simulink model "ThreeDof_2015_11_21"  (R2013a)
settings: Solver=ode45  StartTime=0.0  StopTime=100  RelTol=1e-3
undefined symbols (not defined in the file): cbar, Earth, F, Light, MIL, MSSN, statdyn, WGS84
libraries: aerolibwind2 x3, aerolibtransform2 x3, aerolibasang x3, aerolibactuator x3, aerolibobsolete x2, aerolibconvert2 x2, aerolibatmos2 x1, PowerFlowLib x1, simulink x1, aerolib3dof2 x1, aerolibadyn x1
settings Model: Creator=mwillms4  LastModifiedBy=ASELab1

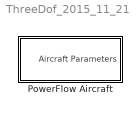
== system ThreeDof_2015_11_21 ==
  PowerFlow Aircraft : Subsystem

== system ThreeDof_2015_11_21/PowerFlow Aircraft ==
  Bus Selector : BusSelector  OutputSignals=alt
  Environment : Subsystem  TreatAsAtomicUnit=on
  Mission Profile : PowerFlowLib/Mission Profile/Mission Profile  mssn_check=off  mssn_prof=MSSN  del_P=0  del_T=0  del_rho=0  pres_msl=101.3  temp_msl=15  dens_msl=1.229
  Pilot : Subsystem  TreatAsAtomicUnit=on
  Scope : Scope
  Vehicle System Model : Subsystem
  Aircraft Parameters : Outport
  wires:
  Environment/1(Env) -> Vehicle System Model/1(Env)
  Pilot/1(cmd) -> Vehicle System Model/2(Pilot)
  Mission Profile/1 -> Pilot/2(Mission Profile)
  Vehicle System Model/1(PlantData) -> Aircraft Parameters/1, Environment/1(plant), Pilot/1(Aircraft), Bus Selector/1
  Bus Selector/1 -> Scope/1  "<alt>"

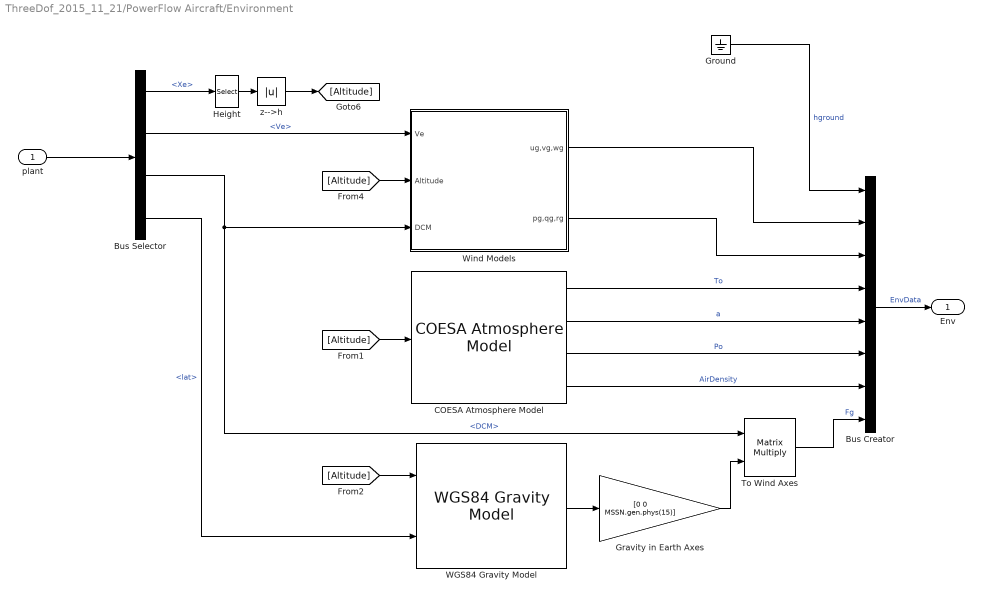
== system ThreeDof_2015_11_21/PowerFlow Aircraft/Environment ==
  plant : Inport
  Bus Creator : BusCreator  Inputs='hground','WindVelocity','WindAngularRates','To','a','Po','AirDensity','Fg'
  Bus Selector : BusSelector  OutputSignals=Xe,Ve,DCM,lat
  COESA Atmosphere Model : aerolibatmos2/COESA Atmosphere Model  units=Metric (MKS)  spec=1976 COESA-extended U.S. Standard Atmosphere  model=Profile  profile_var=High temperature  profile_percent=1%  profile_alt=5 km (16404 ft)  envelope_var=High temperature  envelope_percent=1%  action=Warning
  Gravity in Earth Axes : Gain  Gain=[0 0 MSSN.gen.phys(15)]  SaturateOnIntegerOverflow=on  OutDataTypeStr=Inherit: Same as input  ParamDataTypeStr=Inherit: Same as input
  Ground : Ground
  Height : Selector  IndexMode=Zero-based  InputPortWidth=3  IndexOptions=Index vector (dialog)  Indices=2  OutputSizes=1
  To Wind Axes : Product  Multiplication=Matrix(*)  SaturateOnIntegerOverflow=on  InputSameDT=on  OutDataTypeStr=Inherit: Same as first input
  WGS84 Gravity Model : aerolibobsolete/WGS84 Gravity Model  model=WGS84 Taylor Series  units=Metric (MKS)  no_atmos=on  precessing=on  month=February  day=1  year=2000  no_centrifugal=on  action=Warning
  Wind Models : Subsystem
  z-->h : Abs  SaturateOnIntegerOverflow=on
  Env : Outport  InitialOutput=0
  wires:
  Bus Selector/3 -> Wind Models/3(DCM), To Wind Axes/1  "<DCM>"
  Bus Selector/2 -> Wind Models/1(Ve)  "<Ve>"
  Bus Selector/1 -> Height/1  "<Xe>"
  [Altitude] -> COESA Atmosphere Model/1
  [Altitude] -> WGS84 Gravity Model/1
  [Altitude] -> Wind Models/2(Altitude)
  z-->h/1 -> [Altitude]
  plant/1 -> Bus Selector/1
  Bus Creator/1 -> Env/1  "EnvData"
  To Wind Axes/1 -> Bus Creator/8  "Fg"
  Gravity in Earth Axes/1 -> To Wind Axes/2
  WGS84 Gravity Model/1 -> Gravity in Earth Axes/1
  Bus Selector/4 -> WGS84 Gravity Model/2  "<lat>"
  Height/1 -> z-->h/1
  COESA Atmosphere Model/1 -> Bus Creator/4  "To"
  COESA Atmosphere Model/3 -> Bus Creator/6  "Po"
  COESA Atmosphere Model/2 -> Bus Creator/5  "a"
  COESA Atmosphere Model/4 -> Bus Creator/7  "AirDensity"
  Wind Models/2(pg,qg,rg) -> Bus Creator/3
  Wind Models/1(ug,vg,wg) -> Bus Creator/2
  Ground/1 -> Bus Creator/1  "hground"

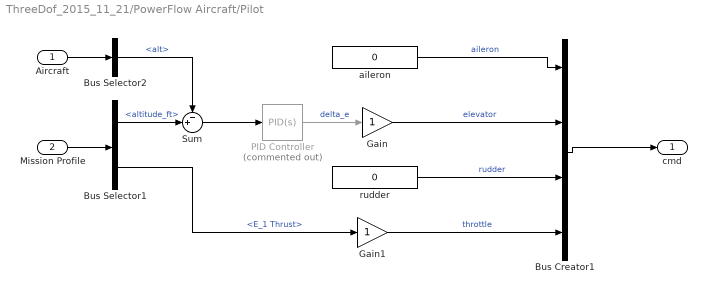
== system ThreeDof_2015_11_21/PowerFlow Aircraft/Pilot ==
  Aircraft : Inport
  Mission Profile : Inport  Port=2
  Bus Creator1 : BusCreator
  Bus Selector1 : BusSelector  OutputSignals=Flight parameters.altitude_ft,Engines.E_1 Thrust
  Bus Selector2 : BusSelector  OutputSignals=alt
  Gain : Gain
  Gain1 : Gain
  PID Controller : simulink/Continuous/PID Controller  Commented=on  Controller=PID  TimeDomain=Continuous-time  SampleTime=1  IntegratorMethod=Forward Euler  FilterMethod=Forward Euler  Form=Parallel  P=1  I=1  D=0  N=100  InitialConditionSource=internal  InitialConditionForIntegrator=0  InitialConditionForFilter=0  ExternalReset=none  LimitOutput=off  UpperSaturationLimit=inf  LowerSaturationLimit=-inf  LinearizeAsGain=on  AntiWindupMode=none  Kb=1  TrackingMode=off  Kt=1  PParamMin=[]  PParamMax=[]  IParamMin=[]  IParamMax=[]  DParamMin=[]  DParamMax=[]  NParamMin=[]  NParamMax=[]  KbParamMin=[]  KbParamMax=[]  KtParamMin=[]  KtParamMax=[]  POutMin=[]  POutMax=[]  IOutMin=[]  IOutMax=[]  DOutMin=[]  DOutMax=[]  NOutMin=[]  NOutMax=[]  KbOutMin=[]  KbOutMax=[]  KtOutMin=[]  KtOutMax=[]  IntegratorOutMin=[]  IntegratorOutMax=[]  FilterOutMin=[]  FilterOutMax=[]  SumOutMin=[]  SumOutMax=[]  SumI1OutMin=[]  SumI1OutMax=[]  SumI2OutMin=[]  SumI2OutMax=[]  SumI3OutMin=[]  SumI3OutMax=[]  SumDOutMin=[]  SumDOutMax=[]  SaturationOutMin=[]  SaturationOutMax=[]  IntegratorContinuousStateAttributes=''  IntegratorStateMustResolveToSignalObject=off  IntegratorRTWStateStorageClass=Auto  FilterContinuousStateAttributes=''  FilterStateMustResolveToSignalObject=off  FilterRTWStateStorageClass=Auto
  Sum : Sum  Inputs=-+|
  aileron : Constant  Value=0  OutDataTypeStr=double
  rudder : Constant  Value=0  OutDataTypeStr=double
  cmd : Outport
  wires:
  PID Controller/1 -> Gain/1  "delta_e"
  aileron/1 -> Bus Creator1/1  "aileron"
  Gain1/1 -> Bus Creator1/4  "throttle"
  rudder/1 -> Bus Creator1/3  "rudder"
  Bus Creator1/1 -> cmd/1
  Mission Profile/1 -> Bus Selector1/1
  Aircraft/1 -> Bus Selector2/1
  Gain/1 -> Bus Creator1/2  "elevator"
  Bus Selector2/1 -> Sum/1  "<alt>"
  Bus Selector1/1 -> Sum/2  "<altitude_ft>"
  Bus Selector1/2 -> Gain1/1  "<E_1 Thrust>"
  Sum/1 -> PID Controller/1

== system ThreeDof_2015_11_21/PowerFlow Aircraft/Vehicle System Model ==
  Env : Inport
  Pilot : Inport  Port=2
  Vehicle : Subsystem
  PlantData : Outport
  wires:
  Env/1 -> Vehicle/1(Env)
  Vehicle/1(AircraftData) -> PlantData/1
  Pilot/1 -> Vehicle/2(Pilot)

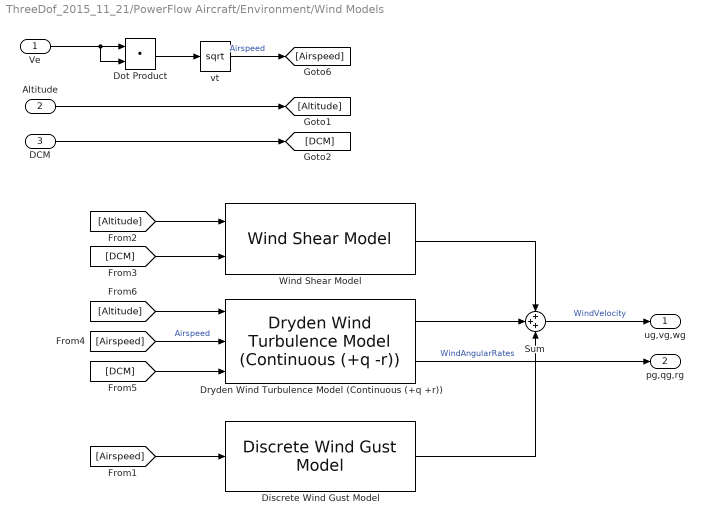
== system ThreeDof_2015_11_21/PowerFlow Aircraft/Environment/Wind Models ==
  Ve : Inport
  Altitude : Inport  Port=2
  DCM : Inport  Port=3
  Discrete Wind Gust Model : aerolibwind2/Discrete Wind Gust Model  units=Metric (MKS)  Gx=off  Gy=off  Gz=off  t_0=20  d_m=[120 120 80]  v_m=[3.5 3.0 3.0]
  Dot Product : DotProduct  OutDataTypeStr=Inherit: Inherit via internal rule
  Dryden Wind Turbulence Model (Continuous (+q +r)) : aerolibwind2/Dryden Wind Turbulence Model  (Continuous (+q -r))  units=Metric (MKS)  spec=MIL-F-8785C  model=Continuous Dryden (+q +r)  W20=5  Wdeg=0  TurbProb=10^-2 - Light  L_high=533.4  Wingspan=4  ts=0.1  Seed=[23341 23342 23343 23344]  T_on=off
  Sum : Sum  Inputs=+++  SaturateOnIntegerOverflow=on  InputSameDT=on  OutDataTypeStr=Inherit: Same as first input
  Wind Shear Model : aerolibwind2/Wind Shear Model  units=Metric (MKS)  phase=Category C - Terminal Flight Phase  W_20=1  Wdeg=0
  vt : Sqrt  SaturateOnIntegerOverflow=on
  ug,vg,wg : Outport
  pg,qg,rg : Outport  Port=2
  wires:
  [Altitude] -> Dryden Wind Turbulence Model (Continuous (+q +r))/1
  [DCM] -> Dryden Wind Turbulence Model (Continuous (+q +r))/3
  [DCM] -> Wind Shear Model/2
  DCM/1 -> [DCM]
  [Altitude] -> Wind Shear Model/1
  Altitude/1 -> [Altitude]
  [Airspeed] -> Discrete Wind Gust Model/1
  vt/1 -> [Airspeed]  "Airspeed"
  Dot Product/1 -> vt/1
  Dryden Wind Turbulence Model (Continuous (+q +r))/2 -> pg,qg,rg/1  "WindAngularRates"
  [Airspeed] -> Dryden Wind Turbulence Model (Continuous (+q +r))/2  "Airspeed"
  Sum/1 -> ug,vg,wg/1  "WindVelocity"
  Discrete Wind Gust Model/1 -> Sum/3
  Dryden Wind Turbulence Model (Continuous (+q +r))/1 -> Sum/2
  Wind Shear Model/1 -> Sum/1
  Ve/1 -> Dot Product/2, Dot Product/1

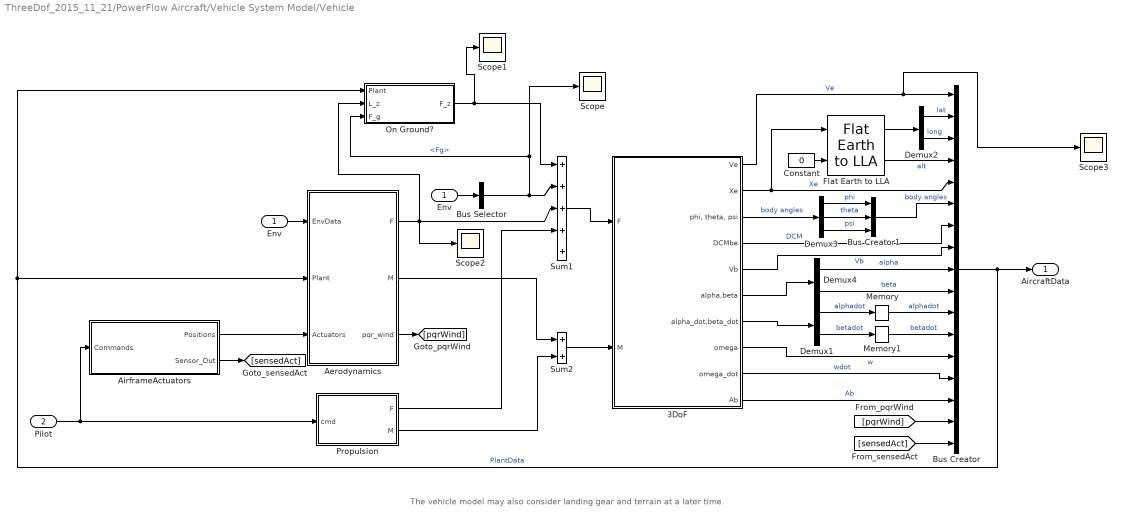
== system ThreeDof_2015_11_21/PowerFlow Aircraft/Vehicle System Model/Vehicle ==
  note: The vehicle model may also consider landing gear and terrain at a later time.
  Env : Inport
  Pilot : Inport  Port=2
  3DoF : Subsystem
  Aerodynamics : Subsystem
  AirframeActuators : Subsystem
  Bus Creator : BusCreator  Inputs=17
  Bus Creator1 : BusCreator  Inputs=3
  Bus Selector : BusSelector  OutputSignals=Fg
  Constant : Constant  Value=0
  Demux1 : Demux  Outputs=2
  Demux2 : Demux  Outputs=2
  Demux3 : Demux  Outputs=3
  Demux4 : Demux  Outputs=2
  "Env " : InportShadow
  Flat Earth to LLA : aerolibtransform2/Flat Earth to LLA  units=Metric (MKS)  ptype=Earth (WGS84)  F=1/298.257223563  R=6378137  LL0=[40.112025 -88.225628]  psi=MSSN.gen.phys(3)
  Memory : Memory  LinearizeMemory=on
  Memory1 : Memory  LinearizeMemory=on
  On Ground? : Subsystem
  Propulsion : Subsystem
      settings: RTWSystemCode=Inline
  Scope{,1..3} (4 alike) : Scope
      Scope settings: ShowLegends=on  YMin=-2.75e+06  YMax=2.75e+06
      Scope1 settings: SaveName=ScopeData2
      Scope2 settings: SaveName=ScopeData3
      Scope3 settings: SaveName=ScopeData4
  Sum1 : Sum  Inputs=+++++  SaturateOnIntegerOverflow=on  InputSameDT=on  OutDataTypeStr=Inherit: Same as first input
  Sum2 : Sum  SaturateOnIntegerOverflow=on  InputSameDT=on  OutDataTypeStr=Inherit: Same as first input
  AircraftData : Outport
  wires:
  Sum1/1 -> 3DoF/1(F)
  Sum2/1 -> 3DoF/2(M)
  3DoF/4(DCMbe) -> Bus Creator/7  "DCM"
  3DoF/5(Vb) -> Bus Creator/8  "Vb"
  3DoF/6(alpha,beta) -> Demux4/1
  3DoF/7(alpha_dot,beta_dot) -> Demux1/1
  3DoF/9(omega_dot) -> Bus Creator/14  "wdot"
  3DoF/10(Ab) -> Bus Creator/15  "Ab"
  Bus Creator/1 -> On Ground?/1(Plant), Aerodynamics/2(Plant), AircraftData/1  "PlantData"
  Aerodynamics/2(M) -> Sum2/1
  Propulsion/1(F) -> Sum1/4
  Propulsion/2(M) -> Sum2/2
  Bus Selector/1 -> Scope/1, On Ground?/3(F_g), Sum1/2  "<Fg>"
  Env/1 -> Aerodynamics/1(EnvData)
  Pilot/1 -> AirframeActuators/1(Commands), Propulsion/1(cmd)
  "Env "/1 -> Bus Selector/1
  AirframeActuators/1(Positions) -> Aerodynamics/3(Actuators)
  Aerodynamics/3(pqr_wind) -> [pqrWind]
  [pqrWind] -> Bus Creator/16
  AirframeActuators/2(Sensor_Out) -> [sensedAct]
  [sensedAct] -> Bus Creator/17
  Constant/1 -> Flat Earth to LLA/2
  Flat Earth to LLA/2 -> Bus Creator/4  "alt"
  Flat Earth to LLA/1 -> Demux2/1
  Demux2/1 -> Bus Creator/2  "lat"
  Demux2/2 -> Bus Creator/3  "long"
  Demux1/1 -> Memory/1  "alphadot"
  Demux1/2 -> Memory1/1  "betadot"
  Demux3/1 -> Bus Creator1/1  "phi"
  Demux3/2 -> Bus Creator1/2  "theta"
  Demux3/3 -> Bus Creator1/3  "psi"
  Bus Creator1/1 -> Bus Creator/6  "body angles"
  3DoF/8(omega) -> Bus Creator/13  "w"
  Demux4/2 -> Bus Creator/10  "beta"
  Demux4/1 -> Bus Creator/9  "alpha"
  Memory/1 -> Bus Creator/11  "alphadot"
  Memory1/1 -> Bus Creator/12  "betadot"
  3DoF/1(Ve) -> Scope3/1, Bus Creator/1  "Ve"
  3DoF/2(Xe) -> Flat Earth to LLA/1, Bus Creator/5  "Xe"
  3DoF/3("phi, theta, psi") -> Demux3/1  "body angles"
  On Ground?/1(F_z) -> Scope1/1, Sum1/1
  Aerodynamics/1(F) -> Scope2/1, On Ground?/2(L_z), Sum1/3

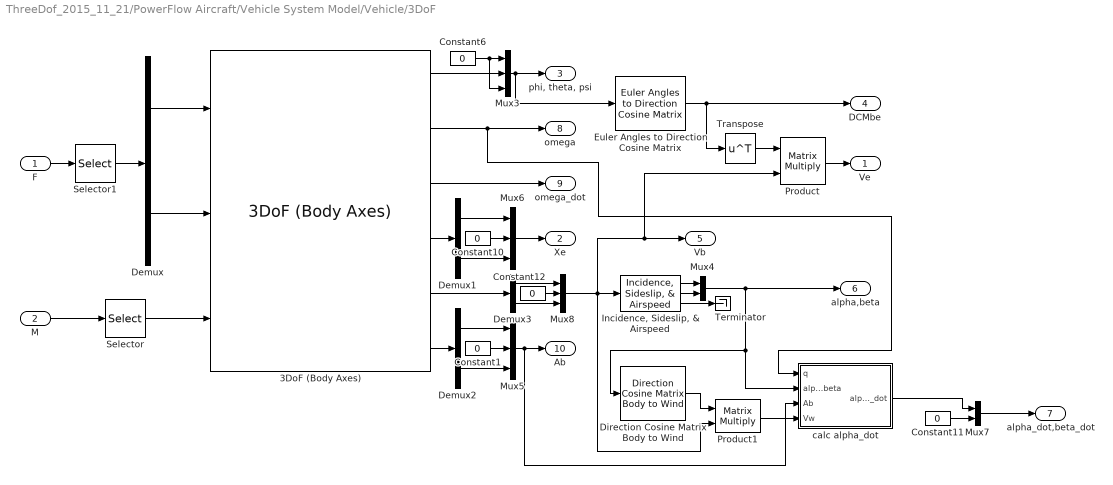
== system ThreeDof_2015_11_21/PowerFlow Aircraft/Vehicle System Model/Vehicle/3DoF ==
  F : Inport
  M : Inport  Port=2
  3DoF (Body Axes) : aerolib3dof2/3DoF (Body Axes)  units=Metric (MKS)  mtype=Fixed  v_ini=0  theta_ini=0  alpha_ini=0  q_ini=0  pos_ini=[0 -MSSN.cond.alt(1)]  mass=MSSN.gen.phys(15)  mass_e=0.5  mass_f=3.0  Iyy=inertia  Iyy_e=0.5  Iyy_f=3.0  g_in=Internal  g=0
  Constant{1,6,10..12} (5 alike) : Constant  Value=0
  Demux{,1..3} (4 alike) : Demux  Outputs=2
  Direction Cosine Matrix Body to Wind : aerolibtransform2/Direction Cosine Matrix Body to Wind
  Euler Angles to Direction Cosine Matrix : aerolibobsolete/Euler Angles to  Direction Cosine Matrix
  "Incidence, Sideslip, & Airspeed" : aerolibasang/Incidence, Sideslip, & Airspeed
  Mux{3,5..6,8} (4 alike) : Mux  Inputs=3
  Mux4 : Mux  Inputs=2
  Mux7 : Mux  Inputs=2
  Product : Product  Multiplication=Matrix(*)  SaturateOnIntegerOverflow=on  InputSameDT=on  OutDataTypeStr=Inherit: Same as first input
  Product1 : Product  Multiplication=Matrix(*)  SaturateOnIntegerOverflow=on  InputSameDT=on  OutDataTypeStr=Inherit: Same as first input
  Selector : Selector  IndexMode=Zero-based  InputPortWidth=3  IndexOptions=Index vector (dialog)  Indices=1  OutputSizes=1
  Selector1 : Selector  IndexMode=Zero-based  InputPortWidth=3  IndexOptions=Index vector (dialog)  Indices=[0 2]  OutputSizes=1
  Terminator : Terminator
  Transpose : Math  Operator=transpose  SaturateOnIntegerOverflow=on
  calc alpha_dot : Subsystem
  Ve : Outport
  Xe : Outport  Port=2
  "phi, theta, psi" : Outport  Port=3
  DCMbe : Outport  Port=4
  Vb : Outport  Port=5
  alpha,beta : Outport  Port=6
  alpha_dot,beta_dot : Outport  Port=7
  omega : Outport  Port=8
  omega_dot : Outport  Port=9
  Ab : Outport  Port=10
  wires:
  F/1 -> Selector1/1
  M/1 -> Selector/1
  Selector/1 -> 3DoF (Body Axes)/3
  Selector1/1 -> Demux/1
  3DoF (Body Axes)/3 -> omega_dot/1
  Mux7/1 -> alpha_dot,beta_dot/1
  Euler Angles to Direction Cosine Matrix/1 -> DCMbe/1, Transpose/1
  3DoF (Body Axes)/5 -> Demux3/1
  Demux/1 -> 3DoF (Body Axes)/1
  Mux6/1 -> Xe/1
  Demux1/1 -> Mux6/1
  Demux1/2 -> Mux6/3
  Constant10/1 -> Mux6/2
  3DoF (Body Axes)/4 -> Demux1/1
  Demux2/1 -> Mux5/1
  Demux2/2 -> Mux5/3
  Constant1/1 -> Mux5/2
  3DoF (Body Axes)/6 -> Demux2/1
  "Incidence, Sideslip, & Airspeed"/2 -> Mux4/2
  Demux3/2 -> Mux8/3
  Constant12/1 -> Mux8/2
  Demux3/1 -> Mux8/1
  "Incidence, Sideslip, & Airspeed"/1 -> Mux4/1
  "Incidence, Sideslip, & Airspeed"/3 -> Terminator/1
  Mux4/1 -> alpha,beta/1, calc alpha_dot/2(alpha,beta), Direction Cosine Matrix Body to Wind/1
  Constant6/1 -> Mux3/3, Mux3/1
  Mux3/1 -> "phi, theta, psi"/1, Euler Angles to Direction Cosine Matrix/1
  Transpose/1 -> Product/1
  Mux8/1 -> "Incidence, Sideslip, & Airspeed"/1, Product/2, Vb/1, Product1/2
  3DoF (Body Axes)/1 -> Mux3/2
  Product/1 -> Ve/1
  calc alpha_dot/1(alpha_dot) -> Mux7/1
  Mux5/1 -> Ab/1, calc alpha_dot/3(Ab)
  3DoF (Body Axes)/2 -> calc alpha_dot/1(q), omega/1
  Constant11/1 -> Mux7/2
  Direction Cosine Matrix Body to Wind/1 -> Product1/1
  Product1/1 -> calc alpha_dot/4(Vw)
  Demux/2 -> 3DoF (Body Axes)/2

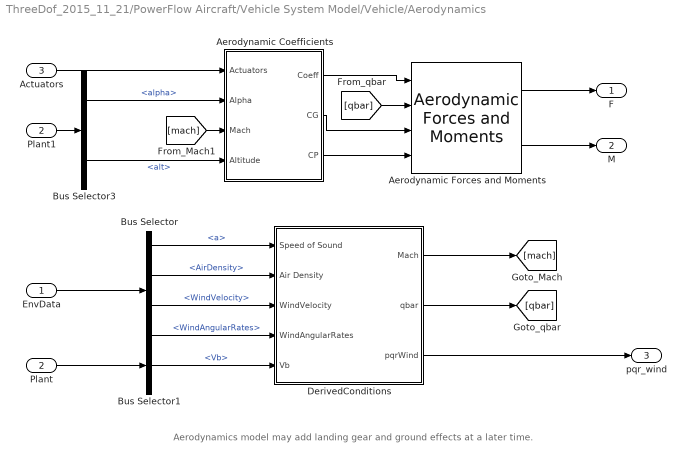
== system ThreeDof_2015_11_21/PowerFlow Aircraft/Vehicle System Model/Vehicle/Aerodynamics ==
  note: Aerodynamics model may add landing gear and ground effects at a later time.
  EnvData : Inport
  Plant : Inport  Port=2
  Actuators : Inport  Port=3
  Aerodynamic Coefficients : Subsystem
  "Aerodynamic Forces and Moments " : aerolibadyn/Aerodynamic Forces and Moments   inputAxes=Body  outputForceAxes=Body  outputMomentAxes=Body  S=MSSN.gen.phys(4)  b=MSSN.gen.phys(5)  cbar=MSSN.gen.phys(6)
  Bus Selector : BusSelector  OutputSignals=a,AirDensity,WindVelocity,WindAngularRates
  Bus Selector1 : BusSelector  OutputSignals=Vb
  Bus Selector3 : BusSelector  OutputSignals=alpha,alt
  DerivedConditions : Subsystem
  Plant1 : InportShadow  Port=2
  F : Outport
  M : Outport  Port=2
  pqr_wind : Outport  Port=3
  wires:
  Aerodynamic Coefficients/1(Coeff) -> "Aerodynamic Forces and Moments "/1
  "Aerodynamic Forces and Moments "/2 -> M/1
  EnvData/1 -> Bus Selector/1
  Bus Selector/1 -> DerivedConditions/1(Speed of Sound)  "<a>"
  Bus Selector/2 -> DerivedConditions/2(Air Density)  "<AirDensity>"
  Bus Selector/3 -> DerivedConditions/3(WindVelocity)  "<WindVelocity>"
  Bus Selector/4 -> DerivedConditions/4(WindAngularRates)  "<WindAngularRates>"
  Plant/1 -> Bus Selector1/1
  Bus Selector1/1 -> DerivedConditions/5(Vb)  "<Vb>"
  Bus Selector3/1 -> Aerodynamic Coefficients/2(Alpha)  "<alpha>"
  DerivedConditions/1(Mach) -> [mach]
  Aerodynamic Coefficients/2(CG) -> "Aerodynamic Forces and Moments "/3
  Aerodynamic Coefficients/3(CP) -> "Aerodynamic Forces and Moments "/4
  DerivedConditions/2(qbar) -> [qbar]
  [qbar] -> "Aerodynamic Forces and Moments "/2
  DerivedConditions/3("pqrWind ") -> pqr_wind/1
  Actuators/1 -> Aerodynamic Coefficients/1(Actuators)
  Bus Selector3/2 -> Aerodynamic Coefficients/4(Altitude)  "<alt>"
  [mach] -> Aerodynamic Coefficients/3(Mach)
  "Aerodynamic Forces and Moments "/1 -> F/1
  Plant1/1 -> Bus Selector3/1

== system ThreeDof_2015_11_21/PowerFlow Aircraft/Vehicle System Model/Vehicle/AirframeActuators ==
  Commands : Inport
  Bus Creator : BusCreator  Inputs=3
  Bus Selector1 : BusSelector  OutputSignals=aileron,elevator,rudder
  Nonlinear Second-Order Actuator : aerolibactuator/Nonlinear Second-Order Actuator  wn_fin=MSSN.gen.phys(7)  z_fin=MSSN.gen.phys(8)  fin_max=MSSN.gen.phys(9)  fin_min=MSSN.gen.phys(12)  fin_maxrate=Inf  fin_act_0=0  fin_act_vel=0
  Nonlinear Second-Order Actuator1 : aerolibactuator/Nonlinear Second-Order Actuator  wn_fin=MSSN.gen.phys(7)  z_fin=MSSN.gen.phys(8)  fin_max=MSSN.gen.phys(10)  fin_min=MSSN.gen.phys(13)  fin_maxrate=Inf  fin_act_0=0  fin_act_vel=0
  Nonlinear Second-Order Actuator2 : aerolibactuator/Nonlinear Second-Order Actuator  wn_fin=MSSN.gen.phys(7)  z_fin=MSSN.gen.phys(8)  fin_max=MSSN.gen.phys(11)  fin_min=MSSN.gen.phys(14)  fin_maxrate=Inf  fin_act_0=0  fin_act_vel=0
  Positions : Outport
  Sensor_Out : Outport  Port=2
  wires:
  Commands/1 -> Bus Selector1/1
  Bus Selector1/1 -> Nonlinear Second-Order Actuator/1  "<aileron>"
  Bus Selector1/2 -> Nonlinear Second-Order Actuator1/1  "<elevator>"
  Bus Selector1/3 -> Nonlinear Second-Order Actuator2/1  "<rudder>"
  Nonlinear Second-Order Actuator2/1 -> Bus Creator/3  "Rudder"
  Bus Creator/1 -> Sensor_Out/1, Positions/1  "Act_positions"
  Nonlinear Second-Order Actuator/1 -> Bus Creator/1  "Aileron"
  Nonlinear Second-Order Actuator1/1 -> Bus Creator/2  "Elevator"

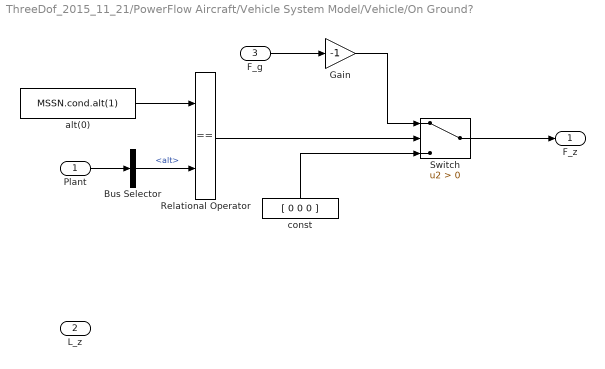
== system ThreeDof_2015_11_21/PowerFlow Aircraft/Vehicle System Model/Vehicle/On Ground? ==
  Plant : Inport
  L_z : Inport  Port=2
  F_g : Inport  Port=3
  Bus Selector : BusSelector  OutputSignals=alt
  Gain : Gain  Gain=-1
  Relational Operator : RelationalOperator  Operator===  OutDataTypeStr=boolean
  Switch : Switch  Criteria=u2 > Threshold
  alt(0) : Constant  Value=MSSN.cond.alt(1)
  const : Constant  Value=[ 0 0 0 ]
  F_z : Outport
  wires:
  Plant/1 -> Bus Selector/1
  Bus Selector/1 -> Relational Operator/2  "<alt>"
  alt(0)/1 -> Relational Operator/1
  Relational Operator/1 -> Switch/2
  F_g/1 -> Gain/1
  Switch/1 -> F_z/1
  const/1 -> Switch/3
  Gain/1 -> Switch/1

== system ThreeDof_2015_11_21/PowerFlow Aircraft/Vehicle System Model/Vehicle/Propulsion ==
  cmd : Inport
  Bus Selector2 : BusSelector  OutputSignals=throttle
  Mux : Mux  Inputs=[1 2]
  ThrustX : Lookup_n-D  NumberOfTableDimensions=1  BreakpointsForDimension1=(1/6)*(3+([-3:3]))  IndexSearchMethod=Linear search  BeginIndexSearchUsingPreviousIndexResult=on  Table=10000*(1+tanh([-3:3]))  ExtrapMethod=Clip  InputSameDT=on
  Thrust_LMN : Constant  Value=[0, 0, 0]  SampleTime=-1
  Thrust_YZ : Constant  Value=[0, 0]  SampleTime=-1
  F : Outport
  M : Outport  Port=2
  wires:
  ThrustX/1 -> Mux/1
  Thrust_YZ/1 -> Mux/2
  Mux/1 -> F/1
  cmd/1 -> Bus Selector2/1
  Thrust_LMN/1 -> M/1
  Bus Selector2/1 -> ThrustX/1  "<throttle>"

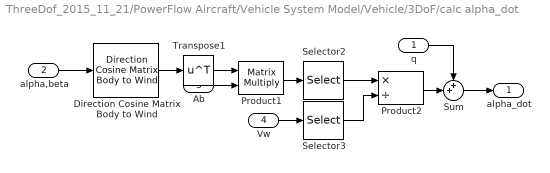
== system ThreeDof_2015_11_21/PowerFlow Aircraft/Vehicle System Model/Vehicle/3DoF/calc alpha_dot ==
  q : Inport
  alpha,beta : Inport  Port=2
  Ab : Inport  Port=3
  Vw : Inport  Port=4
  Direction Cosine Matrix Body to Wind : aerolibtransform2/Direction Cosine Matrix Body to Wind
  Product1 : Product  Multiplication=Matrix(*)  SaturateOnIntegerOverflow=on  InputSameDT=on  OutDataTypeStr=Inherit: Same as first input
  Product2 : Product  Inputs=*/  SaturateOnIntegerOverflow=on  InputSameDT=on  OutDataTypeStr=Inherit: Same as first input
  Selector2 : Selector  IndexMode=Zero-based  InputPortWidth=3  IndexOptions=Index vector (dialog)  Indices=2  OutputSizes=1
  Selector3 : Selector  IndexMode=Zero-based  InputPortWidth=3  IndexOptions=Index vector (dialog)  Indices=0  OutputSizes=1
  Sum : Sum  Inputs=++|
  Transpose1 : Math  Operator=transpose  SaturateOnIntegerOverflow=on
  alpha_dot : Outport
  wires:
  Direction Cosine Matrix Body to Wind/1 -> Transpose1/1
  Transpose1/1 -> Product1/1
  Product1/1 -> Selector2/1
  Selector2/1 -> Product2/1
  Selector3/1 -> Product2/2
  Product2/1 -> Sum/2
  alpha,beta/1 -> Direction Cosine Matrix Body to Wind/1
  q/1 -> Sum/1
  Sum/1 -> alpha_dot/1
  Ab/1 -> Product1/2
  Vw/1 -> Selector3/1

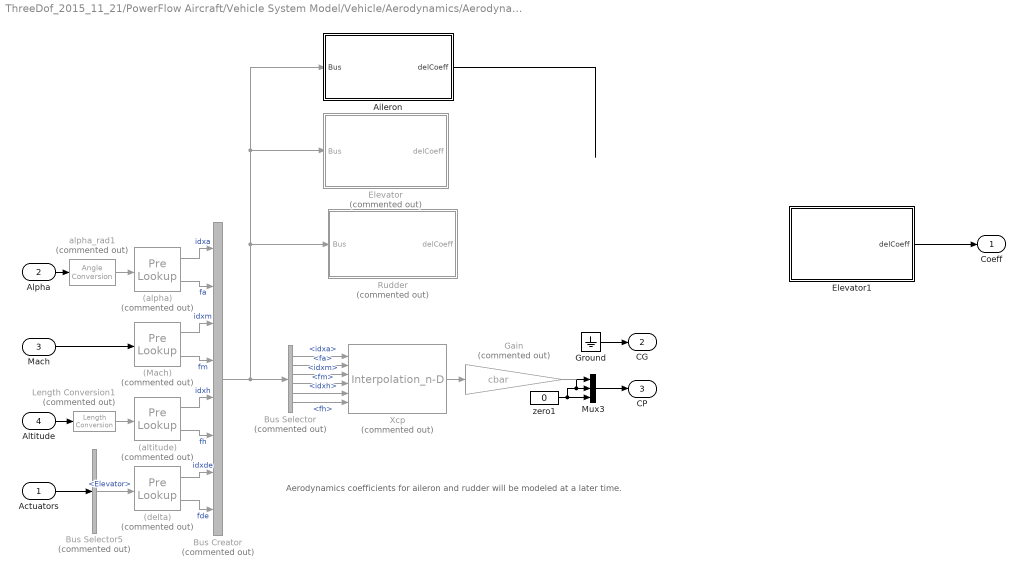
== system ThreeDof_2015_11_21/PowerFlow Aircraft/Vehicle System Model/Vehicle/Aerodynamics/Aerodynamic Coefficients ==
  note: Aerodynamics coefficients for aileron and rudder will be modeled at a later time.
  Actuators : Inport
  Alpha : Inport  Port=2
  Mach : Inport  Port=3
  Altitude : Inport  Port=4
  (Mach) : PreLookup  Commented=on  BreakpointsData=statdyn{1}.mach  BeginIndexSearchUsingPreviousIndexResult=on  ExtrapMethod=Linear  IndexDataTypeStr=int32  FractionDataTypeStr=double
  (alpha) : PreLookup  Commented=on  BreakpointsData=statdyn{1}.alpha  BeginIndexSearchUsingPreviousIndexResult=on  ExtrapMethod=Linear  IndexDataTypeStr=int32  FractionDataTypeStr=double
  (altitude) : PreLookup  Commented=on  BreakpointsData=statdyn{1}.alt  BeginIndexSearchUsingPreviousIndexResult=on  ExtrapMethod=Linear  IndexDataTypeStr=int32  FractionDataTypeStr=double
  (delta) : PreLookup  Commented=on  BreakpointsData=statdyn{1}.delta  BeginIndexSearchUsingPreviousIndexResult=on  ExtrapMethod=Linear  IndexDataTypeStr=int32  FractionDataTypeStr=double
  Aileron : Subsystem
  Bus Creator : BusCreator  Commented=on  Inputs=8
  Bus Selector : BusSelector  Commented=on  OutputSignals=idxa,fa,idxm,fm,idxh,fh
  Bus Selector5 : BusSelector  Commented=on  OutputSignals=Elevator
  Elevator : Subsystem  Commented=on
  Elevator1 : Subsystem
  Gain : Gain  Commented=on  Gain=cbar
  Ground : Ground
  Length Conversion1 : aerolibconvert2/Length Conversion  Commented=on  IU=m  OU=ft
  Mux3 : Mux  Inputs=3
  Rudder : Subsystem  Commented=on
  Xcp : Interpolation_n-D  Commented=on  NumberOfTableDimensions=3  Table="permute(statdyn{1}.xcp,[1  2  3])"  OutDataTypeStr=double
      settings: InputPortMap=u0,u1,u2,u3,u4,u5
  alpha_rad1 : aerolibconvert2/Angle Conversion  Commented=on  IU=rad  OU=deg
  zero1 : Constant  Value=0
  Coeff : Outport  InitialOutput=0
  CG : Outport  Port=2  PortDimensions=3  InitialOutput=0
  CP : Outport  Port=3  PortDimensions=3  InitialOutput=0
  wires:
  Elevator1/1(delCoeff) -> Coeff/1
  Actuators/1 -> Bus Selector5/1
  Ground/1 -> CG/1
  Mux3/1 -> CP/1
  Xcp/1 -> Gain/1
  zero1/1 -> Mux3/1, Mux3/2, Mux3/3
  Gain/1 -> ?
  (alpha)/2 -> Bus Creator/2  "fa"
  (Mach)/2 -> Bus Creator/4  "fm"
  (altitude)/2 -> Bus Creator/6  "fh"
  (altitude)/1 -> Bus Creator/5  "idxh"
  (Mach)/1 -> Bus Creator/3  "idxm"
  (alpha)/1 -> Bus Creator/1  "idxa"
  Bus Selector/1 -> Xcp/1  "<idxa>"
  Bus Selector/2 -> Xcp/2  "<fa>"
  Bus Selector/3 -> Xcp/3  "<idxm>"
  Bus Selector/4 -> Xcp/4  "<fm>"
  Bus Selector/5 -> Xcp/5  "<idxh>"
  Bus Selector/6 -> Xcp/6  "<fh>"
  Bus Creator/1 -> Bus Selector/1, Elevator/1(Bus), Aileron/1(Bus), Rudder/1(Bus)
  Mach/1 -> (Mach)/1
  Altitude/1 -> Length Conversion1/1
  Length Conversion1/1 -> (altitude)/1
  Alpha/1 -> alpha_rad1/1
  alpha_rad1/1 -> (alpha)/1
  (delta)/1 -> Bus Creator/7  "idxde"
  (delta)/2 -> Bus Creator/8  "fde"
  Bus Selector5/1 -> (delta)/1  "<Elevator>"
  Aileron/1(delCoeff) -> ?

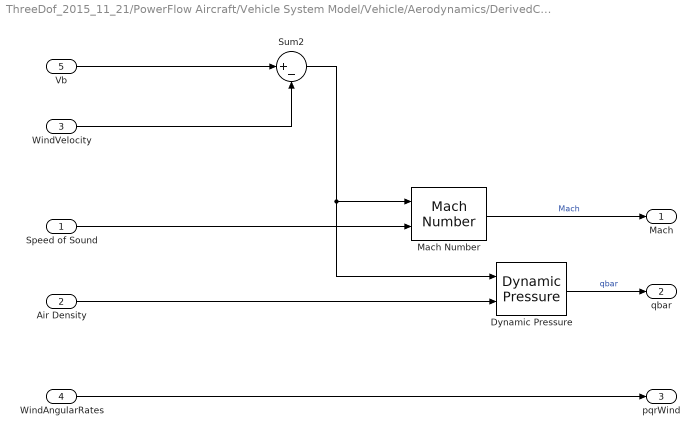
== system ThreeDof_2015_11_21/PowerFlow Aircraft/Vehicle System Model/Vehicle/Aerodynamics/DerivedConditions ==
  Speed of Sound : Inport
  Air Density : Inport  Port=2
  WindVelocity : Inport  Port=3  PortDimensions=3
  WindAngularRates : Inport  Port=4  PortDimensions=3
  Vb : Inport  Port=5  PortDimensions=3
  Dynamic Pressure : aerolibasang/Dynamic Pressure
  Mach Number : aerolibasang/Mach Number
  Sum2 : Sum  Inputs=|+-  SaturateOnIntegerOverflow=on  InputSameDT=on  OutDataTypeStr=Inherit: Same as first input
  Mach : Outport
  qbar : Outport  Port=2  InitialOutput=0
  "pqrWind " : Outport  Port=3
  wires:
  Speed of Sound/1 -> Mach Number/2
  Mach Number/1 -> Mach/1  "Mach"
  Air Density/1 -> Dynamic Pressure/2
  Dynamic Pressure/1 -> qbar/1  "qbar"
  WindAngularRates/1 -> "pqrWind "/1
  Vb/1 -> Sum2/1
  Sum2/1 -> Dynamic Pressure/1, Mach Number/1
  WindVelocity/1 -> Sum2/2

== system ThreeDof_2015_11_21/PowerFlow Aircraft/Vehicle System Model/Vehicle/Aerodynamics/Aerodynamic Coefficients/Aileron ==
  note: Aerodynamics coefficients for aileron and rudder will be modeled at a later time when 6DOF model is developed.
  Bus : Inport
  Constant1 : Constant  Value=0
  Mux1 : Mux  Inputs=6
  Terminator : Terminator
  delCoeff : Outport
  wires:
  Mux1/1 -> delCoeff/1
  Constant1/1 -> Mux1/1, Mux1/2, Mux1/3, Mux1/4, Mux1/5, Mux1/6
  Bus/1 -> Terminator/1

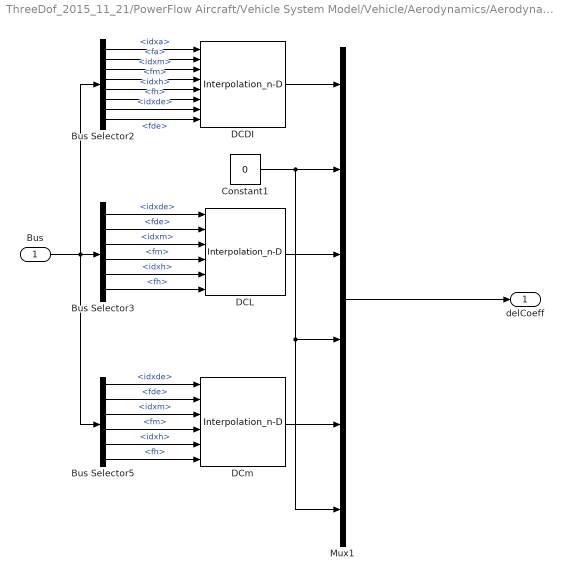
== system ThreeDof_2015_11_21/PowerFlow Aircraft/Vehicle System Model/Vehicle/Aerodynamics/Aerodynamic Coefficients/Elevator ==
  Bus : Inport
  Bus Selector2 : BusSelector  OutputSignals=idxa,fa,idxm,fm,idxh,fh,idxde,fde
  Bus Selector3 : BusSelector  OutputSignals=idxde,fde,idxm,fm,idxh,fh
  Bus Selector5 : BusSelector  OutputSignals=idxde,fde,idxm,fm,idxh,fh
  Constant1 : Constant  Value=0
  DCDI : Interpolation_n-D  NumberOfTableDimensions=4  Table=permute(statdyn{1}.dcdi_sym,[1 3 4 2 ])  RemoveProtectionIndex=on
      settings: InputPortMap=u0,u1,u2,u3,u4,u5,u6,u7
  DCL : Interpolation_n-D  NumberOfTableDimensions=3  Table="permute(statdyn{1}.dcl_sym,[1  2  3])"  RemoveProtectionIndex=on
      settings: InputPortMap=u0,u1,u2,u3,u4,u5
  DCm : Interpolation_n-D  NumberOfTableDimensions=3  Table="permute(statdyn{1}.dcm_sym,[1  2  3])"  RemoveProtectionIndex=on
      settings: InputPortMap=u0,u1,u2,u3,u4,u5
  Mux1 : Mux  Inputs=6
  delCoeff : Outport
  wires:
  Mux1/1 -> delCoeff/1
  Bus/1 -> Bus Selector2/1, Bus Selector3/1, Bus Selector5/1
  DCDI/1 -> Mux1/1
  DCL/1 -> Mux1/3
  DCm/1 -> Mux1/5
  Constant1/1 -> Mux1/2, Mux1/4, Mux1/6
  Bus Selector2/1 -> DCDI/1  "<idxa>"
  Bus Selector2/2 -> DCDI/2  "<fa>"
  Bus Selector3/1 -> DCL/1  "<idxde>"
  Bus Selector3/2 -> DCL/2  "<fde>"
  Bus Selector5/1 -> DCm/1  "<idxde>"
  Bus Selector5/2 -> DCm/2  "<fde>"
  Bus Selector2/3 -> DCDI/3  "<idxm>"
  Bus Selector2/4 -> DCDI/4  "<fm>"
  Bus Selector2/5 -> DCDI/5  "<idxh>"
  Bus Selector2/6 -> DCDI/6  "<fh>"
  Bus Selector2/7 -> DCDI/7  "<idxde>"
  Bus Selector2/8 -> DCDI/8  "<fde>"
  Bus Selector3/3 -> DCL/3  "<idxm>"
  Bus Selector3/4 -> DCL/4  "<fm>"
  Bus Selector3/5 -> DCL/5  "<idxh>"
  Bus Selector3/6 -> DCL/6  "<fh>"
  Bus Selector5/3 -> DCm/3  "<idxm>"
  Bus Selector5/4 -> DCm/4  "<fm>"
  Bus Selector5/5 -> DCm/5  "<idxh>"
  Bus Selector5/6 -> DCm/6  "<fh>"

== system ThreeDof_2015_11_21/PowerFlow Aircraft/Vehicle System Model/Vehicle/Aerodynamics/Aerodynamic Coefficients/Elevator1 ==
  Constant1 : Constant  Value=0
  Constant2 : Constant  Value=0.0164
  Constant3 : Constant  Value=0.21
  Constant4 : Constant  Value=-1.5
  Mux1 : Mux  Inputs=6
  delCoeff : Outport
  wires:
  Constant1/1 -> Mux1/6, Mux1/4, Mux1/2
  Constant4/1 -> Mux1/5
  Constant3/1 -> Mux1/3
  Constant2/1 -> Mux1/1
  Mux1/1 -> delCoeff/1

== system ThreeDof_2015_11_21/PowerFlow Aircraft/Vehicle System Model/Vehicle/Aerodynamics/Aerodynamic Coefficients/Rudder ==
  note: Aerodynamics coefficients for aileron and rudder will be modeled at a later time when 6DOF model is developed.
  Bus : Inport
  Constant1 : Constant  Value=0
  Mux1 : Mux  Inputs=6
  Terminator : Terminator
  delCoeff : Outport
  wires:
  Mux1/1 -> delCoeff/1
  Constant1/1 -> Mux1/6, Mux1/5, Mux1/4, Mux1/3, Mux1/2, Mux1/1
  Bus/1 -> Terminator/1
